simulink model "StaticControl"  (R2015a)
settings: Solver=ode4  StartTime=0.0  StopTime=15  FixedStep=0.001  RelTol=1e-3
values from neighbouring files (symbols this model uses):
  d = 0.15    [Init.m]    (also in KinematicPlot.m; plotVehicle.m)
  D_fixed = [-1;-1]    [Init.m]
  K = 10    [Init.m]
  L = 0.13    [Init.m]    (also in KinematicPlot.m; plotVehicle.m)
  L_e = (1 + err_L)*L    (= 0.13)    [Init.m]
  mode = 0    [Init.m]
  r = 0.1    [Init.m]    (also in KinematicPlot.m)
  R = 2    [Init.m]
  r_e = (1 + err_r)*r    (= 0.1)    [Init.m]
  theta0 = pi    (= 3.14159265359)    [Init.m]
  wd = 0.5    [Init.m]
  x0 = 2.3    [Init.m]
  y0 = 0    [Init.m]
settings Model: Creator=tgvo  LastModifiedBy=tgvo
settings DataIOCC: LimitDataPoints=off

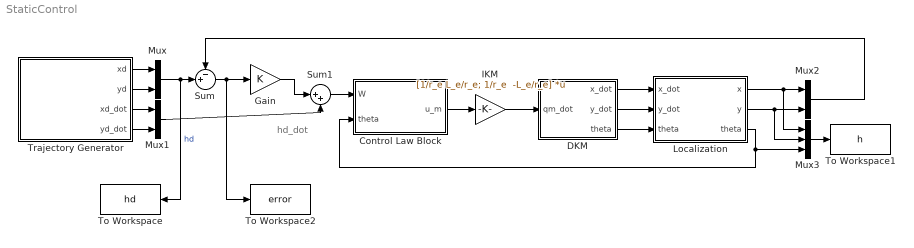
== system StaticControl ==
  note: hd_dot
  Control Law Block : Subsystem  mask{d=d}
      mask prompts: d "Distance between P and Om along x-axis (d)"
  DKM : Subsystem  mask{r=r, L=L, theta0=theta0}
      mask prompts: r "Wheel Raidus (r)"; L "Half of Track Gauge (L)"; theta0 "Initial Theta"
  Gain : Gain  Gain=K
  IKM : Gain  Gain="[1/r_e L_e/r_e; 1/r_e  -L_e/r_e]"  Multiplication=Matrix(K*u) (u vector)
  Localization : Subsystem  mask{x0=x0, y0=y0, d=d}
      mask prompts: x0 "Initial value of x (x0)"; y0 "Initial value of y (y0)"; d "Distance b/w P and Om"
  Mux : Mux  Inputs=2
  Mux1 : Mux  Inputs=2
  Mux2 : Mux  Inputs=2
  Mux3 : Mux  Inputs=3
  Sum : Sum  Inputs=-+|
  Sum1 : Sum  Inputs=|++
  To Workspace : ToWorkspace  VariableName=hd  SampleTime=-1
  To Workspace1 : ToWorkspace  VariableName=h  SampleTime=-1
  To Workspace2 : ToWorkspace  VariableName=error  SampleTime=-1
  Trajectory Generator : Subsystem  mask{R=R, wd=wd, D_fixed=D_fixed, mode=mode}
      mask prompts: R "Radius of Circular Trajectory (R)"; wd "Desired Rotational Velocity (wd)"; D_fixed "Fixed Point"
  wires:
  Trajectory Generator/1(xd) -> Mux/1
  Trajectory Generator/2(yd) -> Mux/2
  Trajectory Generator/3(xd_dot) -> Mux1/1
  Trajectory Generator/4(yd_dot) -> Mux1/2
  Mux/1 -> To Workspace/1, Sum/2  "hd"
  Sum/1 -> To Workspace2/1, Gain/1
  Sum1/1 -> Control Law Block/1(W)
  IKM/1 -> DKM/1(qm_dot)
  Localization/3(theta) -> Mux3/3, Control Law Block/2(theta)
  Localization/1(x) -> Mux3/1, Mux2/1
  Localization/2(y) -> Mux3/2, Mux2/2
  Gain/1 -> Sum1/1
  Mux1/1 -> Sum1/2
  Mux3/1 -> To Workspace1/1
  Mux2/1 -> Sum/1
  DKM/1(x_dot) -> Localization/1(x_dot)
  DKM/2(y_dot) -> Localization/2(y_dot)
  DKM/3(theta) -> Localization/3("theta ")
  Control Law Block/1(u_m) -> IKM/1

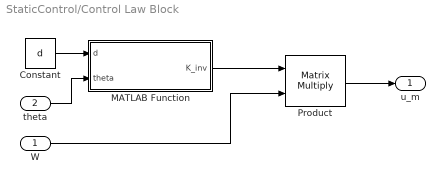
== system StaticControl/Control Law Block ==
  W : Inport
  theta : Inport  Port=2
  Constant : Constant  Value=d
  MATLAB Function : MATLAB Function  TreatAsAtomicUnit=on
  Product : Product  Multiplication=Matrix(*)
  u_m : Outport
  wires:
  theta/1 -> MATLAB Function/2(theta)
  Constant/1 -> MATLAB Function/1(d)
  Product/1 -> u_m/1
  W/1 -> Product/2
  MATLAB Function/1(K_inv) -> Product/1

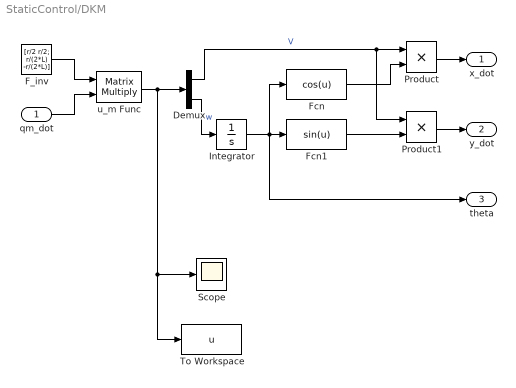
== system StaticControl/DKM ==
  qm_dot : Inport
  Demux : Demux  Outputs=2
  F_inv : Constant  Value=[r/2 r/2; r/(2*L) -r/(2*L)]
  Fcn : Fcn  Expr=cos(u)
  Fcn1 : Fcn  Expr=sin(u)
  Integrator : Integrator  InitialCondition=theta0
  Product : Product
  Product1 : Product
  Scope : Scope
  To Workspace : ToWorkspace  VariableName=u  SampleTime=-1
  u_m Func : Product  Multiplication=Matrix(*)
  x_dot : Outport
  y_dot : Outport  Port=2
  theta : Outport  Port=3
  wires:
  F_inv/1 -> u_m Func/1
  qm_dot/1 -> u_m Func/2
  Demux/2 -> Integrator/1  "w"
  u_m Func/1 -> To Workspace/1, Scope/1, Demux/1
  Fcn/1 -> Product/2
  Fcn1/1 -> Product1/2
  Integrator/1 -> theta/1, Fcn/1, Fcn1/1
  Demux/1 -> Product1/1, Product/1  "V"
  Product/1 -> x_dot/1
  Product1/1 -> y_dot/1

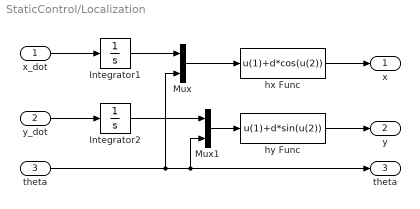
== system StaticControl/Localization ==
  x_dot : Inport
  y_dot : Inport  Port=2
  "theta " : Inport  Port=3
  Integrator1 : Integrator  InitialCondition=x0
  Integrator2 : Integrator  InitialCondition=y0
  Mux : Mux  Inputs=2
  Mux1 : Mux  Inputs=2
  hx Func : Fcn  Expr=u(1)+d*cos(u(2))
  hy Func : Fcn  Expr=u(1)+d*sin(u(2))
  x : Outport
  y : Outport  Port=2
  theta : Outport  Port=3
  wires:
  "theta "/1 -> theta/1, Mux1/2, Mux/2
  x_dot/1 -> Integrator1/1
  y_dot/1 -> Integrator2/1
  hx Func/1 -> x/1
  hy Func/1 -> y/1
  Integrator1/1 -> Mux/1
  Mux/1 -> hx Func/1
  Integrator2/1 -> Mux1/1
  Mux1/1 -> hy Func/1

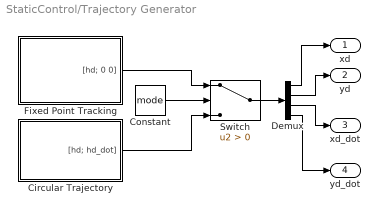
== system StaticControl/Trajectory Generator ==
  Circular Trajectory : Subsystem  mask{R=R, wd=wd}
      mask prompts: R "Circular Radius"; wd "Desired Angular Velocity"
  Constant : Constant  Value=mode
  Demux : Demux
  Fixed Point Tracking : Subsystem  mask{D_fixed=D_fixed}
      mask prompts: D_fixed "Fixed Point"
  Switch : Switch  Criteria=u2 > Threshold
  xd : Outport
  yd : Outport  Port=2
  xd_dot : Outport  Port=3
  yd_dot : Outport  Port=4
  wires:
  Demux/1 -> xd/1
  Demux/2 -> yd/1
  Demux/3 -> xd_dot/1
  Demux/4 -> yd_dot/1
  Constant/1 -> Switch/2
  Circular Trajectory/1("[hd; hd_dot]") -> Switch/3
  Fixed Point Tracking/1("[hd; 0 0]") -> Switch/1
  Switch/1 -> Demux/1

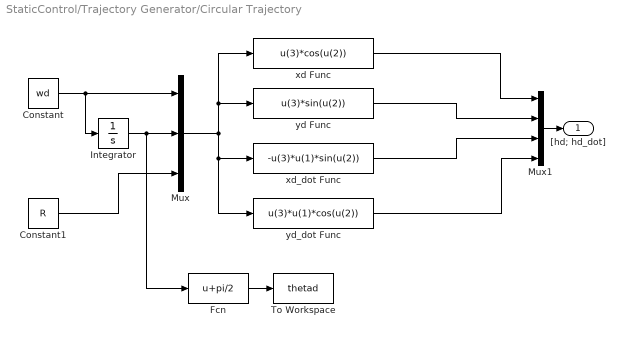
== system StaticControl/Trajectory Generator/Circular Trajectory ==
  Constant : Constant  Value=wd
  Constant1 : Constant  Value=R
  Fcn : Fcn  Expr=u+pi/2
  Integrator : Integrator
  Mux : Mux  Inputs=3
  Mux1 : Mux
  To Workspace : ToWorkspace  VariableName=thetad  SampleTime=-1
  xd Func : Fcn  Expr=u(3)*cos(u(2))
  xd_dot Func : Fcn  Expr=-u(3)*u(1)*sin(u(2))
  yd Func : Fcn  Expr=u(3)*sin(u(2))
  yd_dot Func : Fcn  Expr=u(3)*u(1)*cos(u(2))
  "[hd; hd_dot]" : Outport
  wires:
  Constant1/1 -> Mux/3
  Mux/1 -> yd_dot Func/1, xd_dot Func/1, yd Func/1, xd Func/1
  yd_dot Func/1 -> Mux1/4
  xd Func/1 -> Mux1/1
  xd_dot Func/1 -> Mux1/3
  yd Func/1 -> Mux1/2
  Constant/1 -> Integrator/1, Mux/1
  Integrator/1 -> Fcn/1, Mux/2
  Mux1/1 -> "[hd; hd_dot]"/1
  Fcn/1 -> To Workspace/1

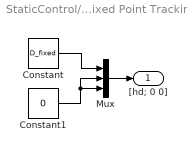
== system StaticControl/Trajectory Generator/Fixed Point Tracking ==
  Constant : Constant  Value=D_fixed
  Constant1 : Constant  Value=0
  Mux : Mux  Inputs=3
  "[hd; 0 0]" : Outport
  wires:
  Constant/1 -> Mux/1
  Constant1/1 -> Mux/3, Mux/2
  Mux/1 -> "[hd; 0 0]"/1

== matlab function StaticControl/Control Law Block/MATLAB Function ==
  data: d input; K_inv output; theta input
function K_inv = Find_K_Inv(d,theta)

K_inv = inv([cos(theta) -d*sin(theta); sin(theta) d*cos(theta)]);
end
